simulink model "MSE312_Lab4_Ex4_3"  (R2023a)
settings: Solver=ode5  StartTime=0.0  StopTime=inf  FixedStep=.01  RelTol=1e-3  EnableMultiTasking=on
libraries: arduinolib x2, slpidlib x1, simulink x1, arduinosensorlib x1, RASPlib x1, robotcorelib x1
settings Model: ExtModeTrigDuration=2  Creator=mwa140  LastModifiedBy=mwa140
settings OptimizationCC: EnhancedBackFolding=on  PassReuseOutputArgsAs=Individual arguments  ZeroExternalMemoryAtStartup=off  ZeroInternalMemoryAtStartup=off  MaxStackSize=64  OptimizeBlockOrder=speed  DifferentSizesBufferReuse=on  OptimizationCustomize=off  EfficientTunableParamExpr=on
settings DebuggingCC: ParameterTunabilityLossMsg=error
settings HardwareCC: ProdBitPerInt=16  ProdBitPerPointer=16  ProdBitPerSizeT=16  ProdBitPerPtrDiffT=16  ProdLargestAtomicFloat=None  ProdWordSize=8  ProdHWDeviceType=Atmel->AVR
settings SFSimCC: MATLABDynamicMemAlloc=off
settings RTWCC: Description=Embedded Coder  SystemTargetFile=ert.tlc  HardwareBoard=Arduino Mega 2560  TemplateMakefile=ert_default_tmf  Toolchain=Arduino AVR  BuildConfiguration=Faster Runs
settings CodeAppCC: ForceParamTrailComments=on  IgnoreCustomStorageClasses=off  OperatorAnnotations=on  SimulinkDataObjDesc=on  SFDataObjDesc=on  InsertBlockDesc=on
settings ERTTargetCC: SupportContinuousTime=on  SupportVariableSizeSignals=on  ExtModeTransport=3  ExtModeStaticAlloc=on  ExtModeAutomaticAllocSize=off  ExtModeStaticAllocSize=2048  ExtModeMexFile=ext_xcp  ExtModeIntrfLevel=Level2 - Open

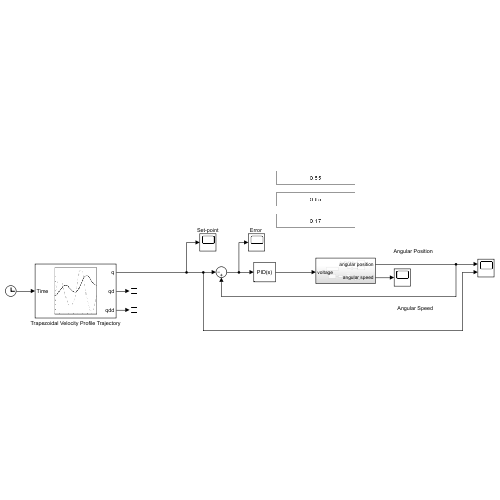
[thumbnail: Simulink's stored preview of the top-level diagram]
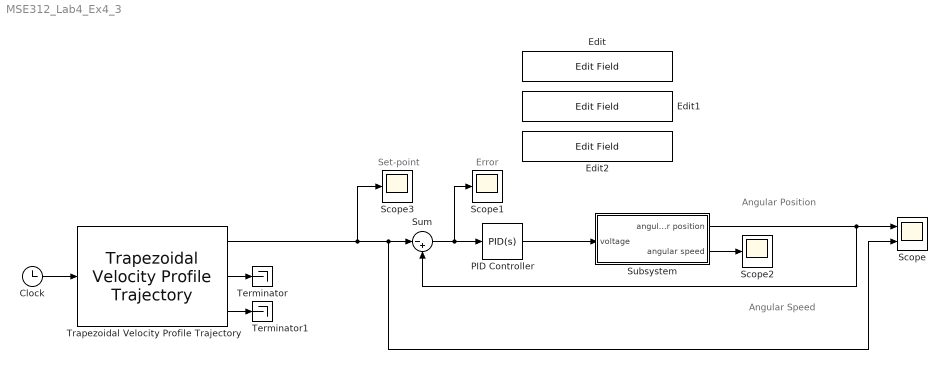
== system MSE312_Lab4_Ex4_3 ==
  note: Set-point
  note: Angular Speed
  note: Angular Position
  note: Error
  Clock : Clock
  Edit : EditField  LabelPosition=Hide  ShowInitialText=on  Alignment=Center
  Edit1 : EditField  LabelPosition=Hide  ShowInitialText=on  Alignment=Center
  Edit2 : EditField  LabelPosition=Hide  ShowInitialText=on  Alignment=Center
  PID Controller : slpidlib/PID Controller  Controller=PID  Form=Parallel  TimeDomain=Continuous-time  UseExternalTs=off  SampleTime=-1  IntegratorMethod=Forward Euler  FilterMethod=Forward Euler  ControllerParametersSource=internal  P=.55  I=.65  UseKiTs=off  D=.17  N=100  UseFilter=on  TunerSelectOption=Transfer Function Based (PID Tuner App)  InitialConditionSource=internal  InitialConditionForIntegrator=0  InitialConditionForFilter=0  DifferentiatorICPrevScaledInput=0  ExternalReset=none  TrackingMode=off  Kt=1  LimitOutput=off  SatLimitsSource=internal  UpperSaturationLimit=inf  LowerSaturationLimit=-inf  LinearizeAsGain=on  AntiWindupMode=none  Kb=1  LimitIntegrator=off  UpperIntegratorSaturationLimit=inf  LowerIntegratorSaturationLimit=-inf  POutMin=[]  POutMax=[]  IOutMin=[]  IOutMax=[]  DOutMin=[]  DOutMax=[]  NOutMin=[]  NOutMax=[]  SumOutMin=[]  SumOutMax=[]  SaturationOutMin=[]  SaturationOutMax=[]  PParamMin=[]  PParamMax=[]  IParamMin=[]  IParamMax=[]  DParamMin=[]  DParamMax=[]  NParamMin=[]  NParamMax=[]  KbParamMin=[]  KbParamMax=[]  KtParamMin=[]  KtParamMax=[]  KbOutMin=[]  KbOutMax=[]  KtOutMin=[]  KtOutMax=[]  IntegratorOutMin=[]  IntegratorOutMax=[]  FilterOutMin=[]  FilterOutMax=[]  SumI1OutMin=[]  SumI1OutMax=[]  SumI2OutMin=[]  SumI2OutMax=[]  SumI3OutMin=[]  SumI3OutMax=[]  SumI4OutMin=[]  SumI4OutMax=[]  SumDOutMin=[]  SumDOutMax=[]  DifferentiatorOutMin=[]  DifferentiatorOutMax=[]  FilterDiffOutCoefMin=[]  FilterDiffOutCoefMax=[]  ReciprocalOutMin=[]  ReciprocalOutMax=[]  SumDenOutMin=[]  SumDenOutMax=[]  SumNumOutMin=[]  SumNumOutMax=[]  DivideOutMin=[]  DivideOutMax=[]  UdiffTsProdOutMin=[]  UdiffTsProdOutMax=[]  NTsProdOutMin=[]  NTsProdOutMax=[]  UintegralTsProdOutMin=[]  UintegralTsProdOutMax=[]  UngainTsProdOutMin=[]  UngainTsProdOutMax=[]  ClampingZeroOutDataTypeStr=Inherit: Inherit via back propagation  ClampingZeroOutMin=[]  ClampingZeroOutMax=[]  FilterDenConstantOutDataTypeStr=Inherit: Inherit via back propagation  FilterDenConstantOutMin=[]  FilterDenConstantOutMax=[]  PCopyOutDataTypeStr=Inherit: Inherit via back propagation  PCopyOutMin=[]  PCopyOutMax=[]  NCopyOutDataTypeStr=Inherit: Inherit via back propagation  NCopyOutMin=[]  NCopyOutMax=[]  IntegratorContinuousStateAttributes=''  IntegratorStateMustResolveToSignalObject=off  IntegratorRTWStateStorageClass=Auto  FilterContinuousStateAttributes=''  FilterStateMustResolveToSignalObject=off  FilterRTWStateStorageClass=Auto  ParallelPVariant=InternalParameters  IdealPVariant=Disabled  IVariant=InternalParameters  DVariant=InternalParameters  IntegratorVariant=Continuous  SatVariant=Disabled  AWVariant=Passthrough  PCopyVariant=Disabled  TRVariant=Disabled  FdbkBlocksVariant=Forward  IdealPFdbkVariant=Disabled  SatFdbkVariant=Disabled  DerivativeFilterVariant=ContFilter  NVariant=InternalParameters  NCopyVariant=Disabled  FilterICVariant=InternalICsFilter  IntegratorICVariant=InternalICs  ExternalResetVariant=Disabled  TRSumVariant=Passthrough  SumFdbkVariant=Disabled  SumVariant=Sum_PID  TsampFilterVariant=InternalTs  TsampNgainVariant=Passthrough  TsampIntegralVariant=Disabled_SignalSpec  ExternalSaturationOutDataTypeStr=Inherit: Same as second input
  Scope : Scope  NumInputPorts=2
  Scope1 : Scope
  Scope2 : Scope
  Scope3 : Scope
  Subsystem : Subsystem
  Sum : Sum  Inputs=|-+
  Terminator : Terminator
  Terminator1 : Terminator
  Trapezoidal Velocity Profile Trajectory : robotcorelib/Trapezoidal Velocity Profile Trajectory  WaypointSource=Internal  Waypoints=[ 0, 90, 0]  NumParams=1  Parameter1=Peak Velocity  Parameter2=End Time  ParameterSource=Internal  PeakVelocity=20  Acceleration=[ 1; 2 ]  EndTime=[ 1; 1 ]  AccelTime=[ 1; 2 ]  SimulateUsing=Interpreted execution
  wires:
  Trapezoidal Velocity Profile Trajectory/2 -> Terminator/1
  Trapezoidal Velocity Profile Trajectory/3 -> Terminator1/1
  Trapezoidal Velocity Profile Trajectory/1 -> Scope3/1, Scope/2, Sum/1
  Clock/1 -> Trapezoidal Velocity Profile Trajectory/1
  Subsystem/2(angular speed) -> Scope2/1
  Sum/1 -> Scope1/1, PID Controller/1
  Subsystem/1(angular position) -> Sum/2, Scope/1
  PID Controller/1 -> Subsystem/1(voltage)

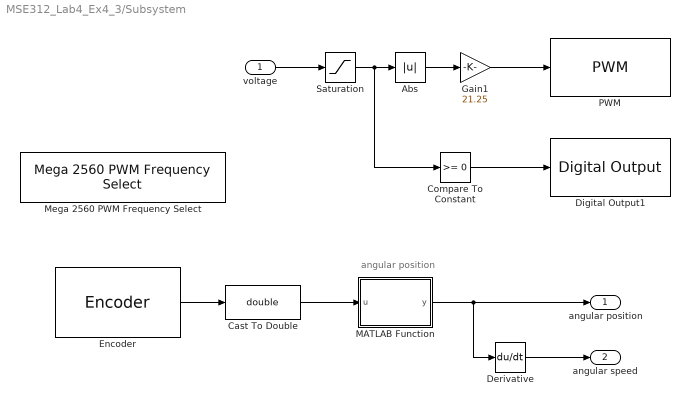
== system MSE312_Lab4_Ex4_3/Subsystem ==
  note: angular position
  voltage : Inport
  Abs : Abs  SaturateOnIntegerOverflow=off
  Cast To Double : DataTypeConversion  OutDataTypeStr=double  SaturateOnIntegerOverflow=off  RndMeth=Floor
  Compare To Constant : simulink/Logic and Bit Operations/Compare To Constant  relop=>=  const=0  OutDataTypeStr=boolean
  Derivative : Derivative  CoefficientInTFapproximation=0.01
  Digital Output1 : arduinolib/Digital Output  pinNumber=10  Direction=output  blockPlatform=arduino
  Encoder : arduinosensorlib/Encoder  InputA=2  InputB=3  Mode=No reset  SampleTime=0.01
  Gain1 : Gain  Gain=21.25
  MATLAB Function : MATLAB Function  TreatAsAtomicUnit=on
  Mega 2560 PWM Frequency Select : RASPlib/Mega 2560 PWM Frequency Select  Frequency=32KHz  Timer=2 - pins 9, 10
      settings: SourceProductName=Rensselaer Arduino Support Package
  PWM : arduinolib/PWM  pinNumber=9  frequencyType=Default  desiredFrequency=490.2  achievableFrequency=490.2
  Saturation : Saturate  UpperLimit=12  LowerLimit=-12
  angular position : Outport
  angular speed : Outport  Port=2
  wires:
  Cast To Double/1 -> MATLAB Function/1(u)
  MATLAB Function/1(y) -> Derivative/1, angular position/1
  Derivative/1 -> angular speed/1
  Saturation/1 -> Compare To Constant/1, Abs/1
  Gain1/1 -> PWM/1
  Abs/1 -> Gain1/1
  Compare To Constant/1 -> Digital Output1/1
  voltage/1 -> Saturation/1
  Encoder/1 -> Cast To Double/1

== matlab function MSE312_Lab4_Ex4_3/Subsystem/MATLAB Function ==
  data: u input; y output
function y = fcn(u)

pos=360/(500*4*6.3);
%pause(1);

y = pos*u;
